simulink model "questao3blocosNlinLinLaplace"  (R2017a)
settings: Solver=VariableStepAuto  StartTime=0.0  StopTime=35  RelTol=1e-3
libraries: simulink x6
settings Model: Creator=julia  LastModifiedBy=julia

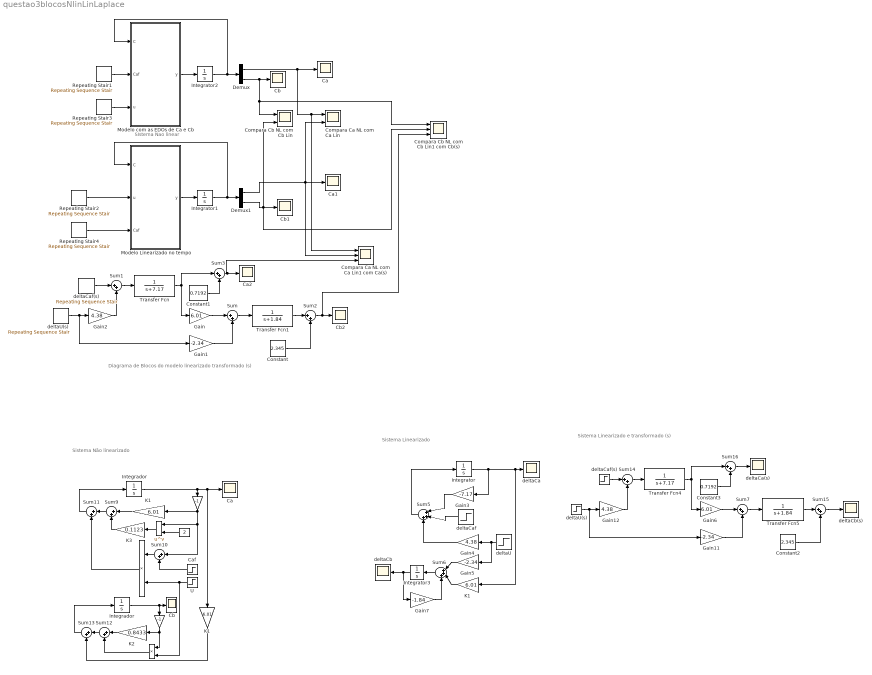
== system questao3blocosNlinLinLaplace ==
  note: Sistema Linearizado
  note: Diagrama de Blocos do modelo linearizado transformado (s)
  note: SIstema Nao linear
  note: Sistema Linearizado e transformado (s)
  note: Sistema Não linearizado
  "   " : Math  Operator=pow  SaturateOnIntegerOverflow=on
  "    " : Constant  Value=2
  "     " : Gain  Gain=-1
  "      " : Product
  "          " : Product
  "               " : Gain  Gain=-1
  Ca : Scope
  "Ca " : Scope
  Ca1 : Scope
  Ca2 : Scope
  Caf : Step  Time=0  After=5.1
  Cb : Scope
  "Cb  " : Scope
  Cb1 : Scope
  Cb2 : Scope
  Compara Cb NL com Cb Lin : Scope  NumInputPorts=2
  Compara Cb NL com Cb Lin1 com Cb(s) : Scope  NumInputPorts=3
  Compara Ca NL com Ca Lin : Scope  NumInputPorts=2
  Compara Ca NL com Ca Lin1 com Ca(s) : Scope  NumInputPorts=3
  Constant : Constant  Value=2.345
  Constant1 : Constant  Value=0.7192
  Constant2 : Constant  Value=2.345
  Constant3 : Constant  Value=0.7192
  Demux : Demux  Outputs=2
  Demux1 : Demux  Outputs=2
  Gain : Gain  Gain=6.01
  Gain1 : Gain  Gain=-2.34
  Gain11 : Gain  Gain=-2.34
  Gain12 : Gain  Gain=4.38
  Gain2 : Gain  Gain=4.38
  Gain3 : Gain  Gain=-7.17
  Gain4 : Gain  Gain=4.38
  Gain5 : Gain  Gain=-2.34
  Gain6 : Gain  Gain=6.01
  Gain7 : Gain  Gain=-1.84
  Integrador : Integrator
  "Integrador " : Integrator
  Integrator : Integrator
  Integrator1 : Integrator  InitialCondition=[0.00001;0.00001]
  Integrator2 : Integrator  InitialCondition=[0.00001;0.00001]
  Integrator3 : Integrator
  K1 : Gain  Gain=6.01
  "K1  " : Gain  Gain=6.01
  "K1   " : Gain  Gain=6.01
  K2 : Gain  Gain=0.8433
  K3 : Gain  Gain=0.1123
  Modelo Linearizado no tempo : MATLAB Function  TreatAsAtomicUnit=on
  Modelo com as EDOs de Ca e Cb : MATLAB Function  TreatAsAtomicUnit=on
  Repeating Stair1 : simulink/Sources/Repeating Sequence Stair  OutValues=[5 5.05 5.10 5.15 5.20]  tsamp=5  OutMin=[]  OutMax=[]  OutDataTypeStr=double  OutputDataTypeScalingMode=double  OutDataType=fixdt(0,8)  ConRadixGroup=Best Precision: Vector-wise  OutScaling=2^-12
  Repeating Stair2 : simulink/Sources/Repeating Sequence Stair  OutValues="[0.90 0.95  1 1.05 1.1]"  tsamp=5  OutMin=[]  OutMax=[]  OutDataTypeStr=double  OutputDataTypeScalingMode=double  OutDataType=fixdt(0,8)  ConRadixGroup=Best Precision: Vector-wise  OutScaling=2^-12
  Repeating Stair3 : simulink/Sources/Repeating Sequence Stair  OutValues="[0.90 0.95  1 1.05 1.1]"  tsamp=5  OutMin=[]  OutMax=[]  OutDataTypeStr=double  OutputDataTypeScalingMode=double  OutDataType=fixdt(0,8)  ConRadixGroup=Best Precision: Vector-wise  OutScaling=2^-12
  Repeating Stair4 : simulink/Sources/Repeating Sequence Stair  OutValues=[5 5.05 5.10 5.15 5.20]  tsamp=5  OutMin=[]  OutMax=[]  OutDataTypeStr=double  OutputDataTypeScalingMode=double  OutDataType=fixdt(0,8)  ConRadixGroup=Best Precision: Vector-wise  OutScaling=2^-12
  Sum{,1..3,7,9..16} (13 alike) : Sum  Inputs=|++
  Sum5 : Sum  Inputs=|+++
  Sum6 : Sum  Inputs=|+++
  Transfer Fcn : TransferFcn  Denominator=[1 7.17]
  Transfer Fcn1 : TransferFcn  Denominator=[1 1.84]
  Transfer Fcn4 : TransferFcn  Denominator=[1 7.17]
  Transfer Fcn5 : TransferFcn  Denominator=[1 1.84]
  U : Step  Time=0
  "deltaCa    " : Scope
  "deltaCa(s)  " : Scope
  "deltaCaf  " : Step  Time=0  After=5.1
  "deltaCaf(s) " : simulink/Sources/Repeating Sequence Stair  OutValues=[0.01 0.05 0.10 0.15 0.20]  tsamp=5  OutMin=[]  OutMax=[]  OutDataTypeStr=double  OutputDataTypeScalingMode=double  OutDataType=fixdt(0,8)  ConRadixGroup=Best Precision: Vector-wise  OutScaling=2^-12
  "deltaCaf(s)  " : Step  Time=40  After=0
  "deltaCb     " : Scope
  "deltaCb(s)  " : Scope
  "deltaU " : Step  Time=40  After=2.345
  deltaU(s) : simulink/Sources/Repeating Sequence Stair  OutValues=[-0.1 -0.05 0 0.05 0.1]  tsamp=5  OutMin=[]  OutMax=[]  OutDataTypeStr=double  OutputDataTypeScalingMode=double  OutDataType=fixdt(0,8)  ConRadixGroup=Best Precision: Vector-wise  OutScaling=2^-12
  "deltaU(s) " : Step  Time=0  After=0
  wires:
  Integrator2/1 -> Demux/1, Modelo com as EDOs de Ca e Cb/1(C)
  Modelo com as EDOs de Ca e Cb/1(y) -> Integrator2/1
  Demux1/1 -> Compara Ca NL com Ca Lin1 com Ca(s)/2, Compara Ca NL com Ca Lin/2, Ca1/1
  Demux1/2 -> Compara Cb NL com Cb Lin/2, Compara Cb NL com Cb Lin1 com Cb(s)/2, Cb1/1
  Modelo Linearizado no tempo/1(y) -> Integrator1/1
  Integrator1/1 -> Modelo Linearizado no tempo/1(C), Demux1/1
  Repeating Stair1/1 -> Modelo com as EDOs de Ca e Cb/2(Caf)
  Repeating Stair3/1 -> Modelo com as EDOs de Ca e Cb/3(u)
  Repeating Stair2/1 -> Modelo Linearizado no tempo/2(u)
  Repeating Stair4/1 -> Modelo Linearizado no tempo/3(Caf)
  Demux/1 -> Ca/1, Compara Ca NL com Ca Lin1 com Ca(s)/1, Compara Ca NL com Ca Lin/1
  Demux/2 -> Compara Cb NL com Cb Lin1 com Cb(s)/1, Compara Cb NL com Cb Lin/1, Cb/1
  Transfer Fcn/1 -> Sum3/1, Gain/1
  Gain/1 -> Sum/1
  Gain1/1 -> Sum/2
  Sum/1 -> Transfer Fcn1/1
  Sum1/1 -> Transfer Fcn/1
  Gain2/1 -> Sum1/2
  deltaU(s)/1 -> Gain1/1, Gain2/1
  "deltaCaf(s) "/1 -> Sum1/1
  Transfer Fcn1/1 -> Sum2/1
  Sum2/1 -> Compara Cb NL com Cb Lin1 com Cb(s)/3, Cb2/1
  Constant/1 -> Sum2/2
  Sum3/1 -> Compara Ca NL com Ca Lin1 com Ca(s)/3, Ca2/1
  Constant1/1 -> Sum3/2
  Sum5/1 -> Integrator/1
  Integrator/1 -> "deltaCa    "/1, K1/1, Gain3/1
  Gain7/1 -> Sum6/3
  Gain5/1 -> Sum6/1
  "deltaCaf  "/1 -> Sum5/2
  Sum6/1 -> Integrator3/1
  Gain3/1 -> Sum5/1
  "deltaU "/1 -> Gain5/1, Gain4/1
  Gain4/1 -> Sum5/3
  Integrator3/1 -> "deltaCb     "/1, Gain7/1
  K1/1 -> Sum6/2
  "   "/1 -> K3/1
  "    "/1 -> "   "/2
  K3/1 -> Sum9/2
  "K1  "/1 -> Sum9/1
  Sum10/1 -> "          "/1
  Sum9/1 -> Sum11/1
  "          "/1 -> Sum11/2
  Sum11/1 -> "Integrador "/1
  K2/1 -> Sum12/1
  "      "/1 -> Sum12/2
  Sum12/1 -> Sum13/1
  "K1   "/1 -> Sum13/2
  Sum13/1 -> Integrador/1
  "     "/1 -> Sum10/1, "   "/1, "K1  "/1
  "               "/1 -> K2/1, "      "/1
  Integrador/1 -> "               "/1, "Cb  "/1
  Caf/1 -> Sum10/2
  U/1 -> "      "/2, "          "/2
  "Integrador "/1 -> "     "/1, "Ca "/1, "K1   "/1
  Constant3/1 -> Sum16/2
  Sum16/1 -> "deltaCa(s)  "/1
  Constant2/1 -> Sum15/2
  Sum15/1 -> "deltaCb(s)  "/1
  Transfer Fcn5/1 -> Sum15/1
  Gain12/1 -> Sum14/2
  Sum14/1 -> Transfer Fcn4/1
  Sum7/1 -> Transfer Fcn5/1
  Gain11/1 -> Sum7/2
  Gain6/1 -> Sum7/1
  Transfer Fcn4/1 -> Gain6/1, Sum16/1
  "deltaU(s) "/1 -> Gain11/1, Gain12/1
  "deltaCaf(s)  "/1 -> Sum14/1

== matlab function questao3blocosNlinLinLaplace/Modelo Linearizado no tempo ==
  data: y output; C input; u input; Caf input
%EDOs das concentracoes dos produtos A e B
function y = fcn(C, u, Caf)

%parametros
k1 = 6.01; %L/min
k2 = 0.8433; %L/min
k3 = 0.1123; %mol/Lmin

%variavel manipulada u = F/V  = [0, 10] L/min = vazao volumetrica
uEq = 1;
%perturbacao Caf = [4, 6] mol/L = concentracao do produto A no fluido de alimentacao
CafEq = 5.1;
%variavel de processo Cb = concentracao do produto B
CbEq = 2.345;
%variavel intermediaria Ca = concentracao do produto A
CaEq = 0.7192;

%variaveis das concentracoes dos produtos A e B
Ca = C(1);
Cb = C(2);

%EDOs linearizadas perto do ponto de equilibrio
Ca_d =  (-k1 - 2*k3*CafEq - uEq)*(Ca - CaEq) + uEq*(Caf - CafEq) + (CafEq - CaEq)*(u   - uEq);
Cb_d=   k1*(Ca - CaEq) + (-k2 - uEq)*(Cb - CbEq) - (CbEq)*(u   - uEq);
 
%conjunto das EDOs
y = [Ca_d;Cb_d];

== matlab function questao3blocosNlinLinLaplace/Modelo com as EDOs de Ca e Cb ==
  data: y output; C input; Caf input; u input
%EDOs das concentracoes dos produtos A e B
function y = fcn(C, Caf, u)

%constantes
k1 = 6.01; %L/min
k2 = 0.8433; %L/min
k3 = 0.1123; %mol/Lmin

%variaveis das concentracoes dos produtos A e B
Ca = C(1);
Cb = C(2);

%EDOs
Ca_d = -k1*Ca - k3*(Ca^2) + (Caf - Ca)*u;
Cb_d =  k1*Ca - k2*Cb - Cb*u;
 
%conjunto das EDOs
y = [Ca_d;Cb_d];
